simulink model "Task_No6_Thermal"  (R2023b)
settings: Solver=ode5  StartTime=0.0  StopTime=3600*24*7  FixedStep=1  RelTol=1e-3
InitFcn:
  | PARAMETERS;
StartFcn:
  | PARAMETERS;
values from neighbouring files (symbols this model uses):
  Conv_C_to_K = 273.15    [PARAMETERS.m]
  P_AC_AIR_FLOW = 1    [PARAMETERS.m]
  P_AREA_BATH = 2*4    (= 8)    [PARAMETERS.m]
  P_AREA_BDR1 = 3.87^2    (= 14.9769)    [PARAMETERS.m]
  P_AREA_BDR2 = 3.87*4.5    (= 17.415)    [PARAMETERS.m]
  P_AREA_EAST_WALL_BATH = 2*P_RM_HEIGHT - P_AREA_WIN_BATH    (= 3.7)    [PARAMETERS.m]
  P_AREA_EAST_WALL_BDR2 = 3.87*P_RM_HEIGHT - P_AREA_WIN_BDRS    (= 7.075)    [PARAMETERS.m]
  P_AREA_EAST_WALL_KIT = 4.13*P_RM_HEIGHT    (= 10.325)    [PARAMETERS.m]
  P_AREA_HALL = 2*6    (= 12)    [PARAMETERS.m]
  P_AREA_KIT = 4.13*4    (= 16.52)    [PARAMETERS.m]
  P_AREA_LVR = 4.13*6    (= 24.78)    [PARAMETERS.m]
  P_AREA_NORTH_WALL_BATH = 1.63*P_RM_HEIGHT    (= 4.075)    [PARAMETERS.m]
  P_AREA_NORTH_WALL_BDR1 = 3.87*P_RM_HEIGHT - P_AREA_WIN_BDRS    (= 7.075)    [PARAMETERS.m]
  P_AREA_NORTH_WALL_BDR2 = 4.5*P_RM_HEIGHT - P_AREA_WIN_BDRS    (= 8.65)    [PARAMETERS.m]
  P_AREA_OUTER_WALL_BATH = (1.63+2)*P_RM_HEIGHT - P_AREA_WIN_BATH    (= 7.775)    [PARAMETERS.m]
  P_AREA_OUTER_WALL_BDR1 = 3.87*2*P_RM_HEIGHT - P_AREA_WIN_BDRS    (= 16.75)    [PARAMETERS.m]
  P_AREA_OUTER_WALL_BDR2 = (4.5+3.87)*P_RM_HEIGHT - P_AREA_WIN_BDRS*2    (= 15.725)    [PARAMETERS.m]
  P_AREA_OUTER_WALL_HALL = 2*P_RM_HEIGHT - P_AREA_SING_DOOR    (= 2.9)    [PARAMETERS.m]
  P_AREA_OUTER_WALL_KIT = (4+4.13)*P_RM_HEIGHT - P_AREA_WIN_KIT    (= 13.725)    [PARAMETERS.m]
  P_AREA_OUTER_WALL_LVR = (4.13+6)*P_RM_HEIGHT - P_AREA_WIN_LVR    (= 14.325)    [PARAMETERS.m]
  P_AREA_SOUTH_WALL_KIT = 4*P_RM_HEIGHT - P_AREA_WIN_KIT    (= 3.4)    [PARAMETERS.m]
  P_AREA_SOUTH_WALL_LVR = 6*P_RM_HEIGHT - P_AREA_WIN_LVR    (= 4)    [PARAMETERS.m]
  P_AREA_WALL_BATH_KIT = 4*P_RM_HEIGHT    (= 10)    [PARAMETERS.m]
  P_AREA_WALL_BDR1_BDR2 = 3.87*P_RM_HEIGHT    (= 9.675)    [PARAMETERS.m]
  P_AREA_WALL_BDR1_HALL = 3.87*P_RM_HEIGHT - P_AREA_SING_DOOR    (= 7.575)    [PARAMETERS.m]
  P_AREA_WALL_BDR2_BATH = 2.37*P_RM_HEIGHT    (= 5.925)    [PARAMETERS.m]
  P_AREA_WALL_BDR2_HALL = 2.13*P_RM_HEIGHT - P_AREA_SING_DOOR    (= 3.225)    [PARAMETERS.m]
  P_AREA_WALL_HALL_BATH = 2*P_RM_HEIGHT - P_AREA_SING_DOOR    (= 2.9)    [PARAMETERS.m]
  P_AREA_WALL_HALL_LVR = 6*P_RM_HEIGHT - P_AREA_DBL_DOOR    (= 10.8)    [PARAMETERS.m]
  P_AREA_WALL_LVR_KIT = 4.13*P_RM_HEIGHT - P_AREA_DBL_DOOR    (= 6.125)    [PARAMETERS.m]
  P_AREA_WIN_BATH = P_H_WIN_NORM*P_W_WIN_BATH    (= 1.3)    [PARAMETERS.m]
  P_AREA_WIN_BDRS = P_H_WIN_NORM*P_W_WIN_BDRS    (= 2.6)    [PARAMETERS.m]
  P_AREA_WIN_KIT = P_H_WIN_DOOR*P_W_WIN_KIT    (= 6.6)    [PARAMETERS.m]
  P_AREA_WIN_LVR = P_H_WIN_DOOR*P_W_WIN_LVR    (= 11)    [PARAMETERS.m]
  P_CP_AIR = 1012    [PARAMETERS.m]
  P_DENSITY_BRICK = 2/(10^-3)    (= 2000)    [PARAMETERS.m]
  P_DENSITY_PUR = 150    [PARAMETERS.m]
  P_EM_GLASS = 0.94    [PARAMETERS.m]
  P_EM_WALL = 0.94    [PARAMETERS.m]
  P_HUMAN = 60    [PARAMETERS.m]
  P_M_WINDOW_SPEC = 20    [PARAMETERS.m]
  P_THICK_BRICK = 0.175    [PARAMETERS.m]
  P_THICK_PUR = P_THICK_WALL - P_THICK_BRICK    (= 0.125)    [PARAMETERS.m]
  T_COOLER = 12    [PARAMETERS.m]
  T_HEATER = 50    [PARAMETERS.m]
  T_INIT_BDR = 22    [PARAMETERS.m]
  T_INIT_OUT = 2.9    [PARAMETERS.m]
  U_CEIL = 1.1    [PARAMETERS.m]
  U_INNER_WALL_BR = 3    [PARAMETERS.m]
  U_INNER_WALL_PC = 0.6    [PARAMETERS.m]
  U_WALL = 0.32    [PARAMETERS.m]
  U_WINDOW = 3.0    (= 3)    [PARAMETERS.m]
undefined symbols (not defined in the file or in its folder): TBL_SOL_EAST_01, TBL_SOL_EAST_02, TBL_SOL_EAST_03, TBL_SOL_EAST_04, TBL_SOL_EAST_05, TBL_SOL_EAST_06, TBL_SOL_EAST_07, TBL_SOL_EAST_08, TBL_SOL_EAST_09, TBL_SOL_EAST_10, TBL_SOL_EAST_11, TBL_SOL_EAST_12, TBL_SOL_NORTH_01, TBL_SOL_NORTH_02, TBL_SOL_NORTH_03, TBL_SOL_NORTH_04, TBL_SOL_NORTH_05, TBL_SOL_NORTH_06, TBL_SOL_NORTH_07, TBL_SOL_NORTH_08, TBL_SOL_NORTH_09, TBL_SOL_NORTH_10, TBL_SOL_NORTH_11, TBL_SOL_NORTH_12, TBL_SOL_SOUTH_01, TBL_TEMP
libraries: fl_lib x135, nesl_utility x39, slpidlib x3
(part 1 of 3)
settings Model: Creator=Selim  LastModifiedBy=Selim

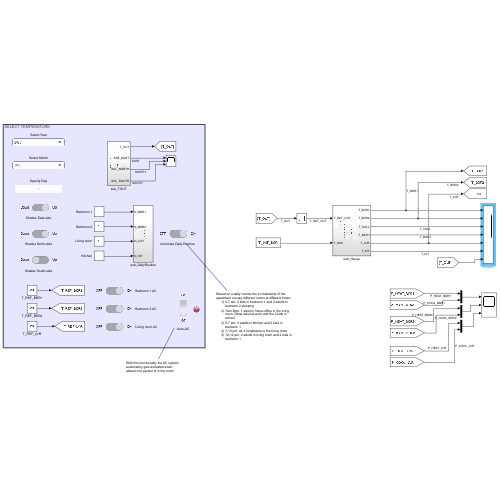
[thumbnail: Simulink's stored preview of the top-level diagram]
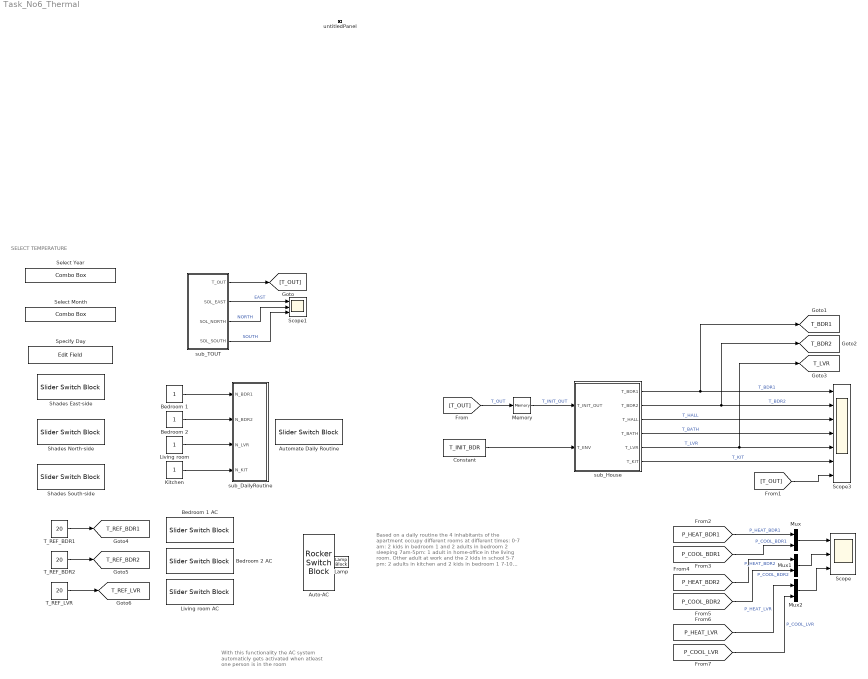
== system Task_No6_Thermal ==
  note: With this functionality the AC system automaticly gets activated when atleast one person is in the room
  note: SELECT TEMPERATURE
  note: Based on a daily routine the 4 inhabitants of the apartment occupy different rooms at different times:
      | 0-7 am: 2 kids in bedroom 1 and 2 adults in bedroom 2 sleeping
      | 7am-5pm: 1 adult in home-office in the living room. Other adult at work and the 2 kids in school
      | 5-7 pm: 2 adults in kitchen and 2 kids in bedroom 1
      | 7-10 pm: all 4 inhabitants in the living room
      | 10-12 pm: 2 adults in living room and 2 kids in bedroom 1
  Auto-AC : RockerSwitchBlock  LabelPosition=Hide
      settings: Values={{'Off', 'On'}, [0 1]}
  Automate Daily Routine : SliderSwitchBlock  LabelPosition=Hide
      settings: Values={{'OFF', 'ON'}, [0 1]}
  Bedroom 1 : Constant
  Bedroom 1 AC : SliderSwitchBlock  LabelPosition=Hide
      settings: Values={{'OFF', 'ON'}, [0 1]}
  Bedroom 2 : Constant
  Bedroom 2 AC : SliderSwitchBlock  LabelPosition=Hide
      settings: Values={{'OFF', 'ON'}, [0 1]}
  Constant : Constant  Value=T_INIT_BDR
  Kitchen : Constant
  Lamp : LampBlock  LabelPosition=Hide
  Living room : Constant
  Living room AC : SliderSwitchBlock  LabelPosition=Hide
      settings: Values={{'OFF', 'ON'}, [0 1]}
  Memory : Memory  InitialCondition=T_INIT_OUT
  Mux : Mux  Inputs=2
  Mux1 : Mux  Inputs=2
  Mux2 : Mux  Inputs=2
  Scope : Scope  NumInputPorts=3
  Scope1 : Scope  NumInputPorts=3
  Scope3 : Scope  NumInputPorts=7
  Select Month : ComboBox  LabelPosition=Hide  SelectedLabel=July
      settings: Values={{'January', 'February', 'March', 'April', 'May', 'June', 'July', 'August', 'September', 'Oktober', 'November', 'December'}, [1 2 3 4 5 6 7 8 9 10 11 12]}
  Select Year : ComboBox  LabelPosition=Hide  SelectedLabel=2023
      settings: Values={{'2022', '2023'}, [2022 2023]}
  Shades East-side : SliderSwitchBlock  LabelPosition=Hide
      settings: Values={{'Down', 'Up'}, [0 1]}
  Shades North-side : SliderSwitchBlock  LabelPosition=Hide
      settings: Values={{'Down', 'Up'}, [0 1]}
  Shades South-side : SliderSwitchBlock  LabelPosition=Hide
      settings: Values={{'Down', 'Up'}, [0 1]}
  Specify Day : EditField  LabelPosition=Hide  ShowInitialText=on  Alignment=Center
  T_REF_BDR1 : Constant  Value=20
  T_REF_BDR2 : Constant  Value=20
  T_REF_LVR : Constant  Value=20
  sub_DailyRoutine : Subsystem
  sub_House : Subsystem
  sub_TOUT : Subsystem
  untitledPanel : Subsystem  Tag=HiddenForWebPanel  IsWebBlockPanel=on
  tag scope: T_BDR1=global, T_BDR2=global, T_LVR=global, T_REF_BDR1=global, T_REF_BDR2=global, T_REF_LVR=global
  wires:
  Memory/1 -> sub_House/1(T_INIT_OUT)  "T_INIT_OUT"
  sub_House/1(T_BDR1) -> [T_BDR1], Scope3/1  "T_BDR1"
  [T_OUT] -> Memory/1  "T_OUT"
  [T_OUT] -> Scope3/7
  Constant/1 -> sub_House/2(T_ENV)
  sub_TOUT/1(T_OUT) -> [T_OUT]
  sub_House/2(T_BDR2) -> [T_BDR2], Scope3/2  "T_BDR2"
  sub_House/3(T_HALL) -> Scope3/3  "T_HALL"
  sub_House/4(T_BATH) -> Scope3/4  "T_BATH"
  sub_House/5(T_LVR) -> [T_LVR], Scope3/5  "T_LVR"
  sub_House/6(T_KIT) -> Scope3/6  "T_KIT"
  sub_TOUT/2(SOL_EAST) -> Scope1/1  "EAST"
  sub_TOUT/3(SOL_NORTH) -> Scope1/2  "NORTH"
  sub_TOUT/4(SOL_SOUTH) -> Scope1/3  "SOUTH"
  Bedroom 1/1 -> sub_DailyRoutine/1(N_BDR1)
  Bedroom 2/1 -> sub_DailyRoutine/2(N_BDR2)
  Living room/1 -> sub_DailyRoutine/3(N_LVR)
  Kitchen/1 -> sub_DailyRoutine/4(N_KIT)
  T_REF_BDR1/1 -> [T_REF_BDR1]
  T_REF_BDR2/1 -> [T_REF_BDR2]
  T_REF_LVR/1 -> [T_REF_LVR]
  Mux/1 -> Scope/1
  Mux1/1 -> Scope/2
  Mux2/1 -> Scope/3
  [P_HEAT_BDR1] -> Mux/1  "P_HEAT_BDR1"
  [P_COOL_BDR1] -> Mux/2  "P_COOL_BDR1"
  [P_HEAT_BDR2] -> Mux1/1  "P_HEAT_BDR2"
  [P_COOL_BDR2] -> Mux1/2  "P_COOL_BDR2"
  [P_HEAT_LVR] -> Mux2/1  "P_HEAT_LVR"
  [P_COOL_LVR] -> Mux2/2  "P_COOL_LVR"

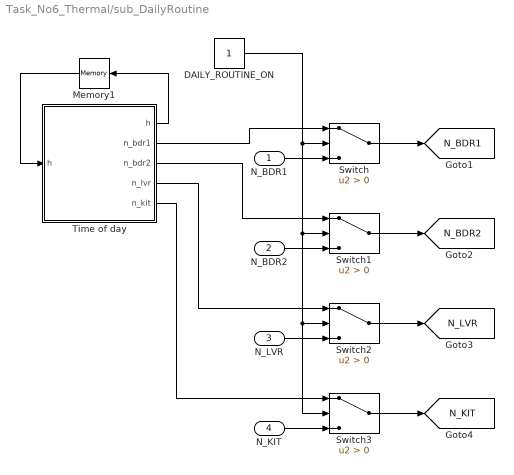
== system Task_No6_Thermal/sub_DailyRoutine ==
  N_BDR1 : Inport
  N_BDR2 : Inport  Port=2
  N_LVR : Inport  Port=3
  N_KIT : Inport  Port=4
  DAILY_ROUTINE_ON : Constant
  Memory1 : Memory
  Switch{,1..3} (4 alike) : Switch  Criteria=u2 > Threshold  SaturateOnIntegerOverflow=off  InputSameDT=off
  Time of day : MATLAB Function  TreatAsAtomicUnit=on
  tag scope: N_BDR1=global, N_BDR2=global, N_KIT=global, N_LVR=global
  wires:
  Switch1/1 -> [N_BDR2]
  Switch2/1 -> [N_LVR]
  Time of day/1(h) -> Memory1/1
  Memory1/1 -> Time of day/1("h ")
  Switch/1 -> [N_BDR1]
  Switch3/1 -> [N_KIT]
  Time of day/2(n_bdr1) -> Switch/1
  Time of day/3(n_bdr2) -> Switch1/1
  Time of day/4(n_lvr) -> Switch2/1
  Time of day/5(n_kit) -> Switch3/1
  DAILY_ROUTINE_ON/1 -> Switch3/2, Switch2/2, Switch1/2, Switch/2
  N_BDR1/1 -> Switch/3
  N_BDR2/1 -> Switch1/3
  N_LVR/1 -> Switch2/3
  N_KIT/1 -> Switch3/3

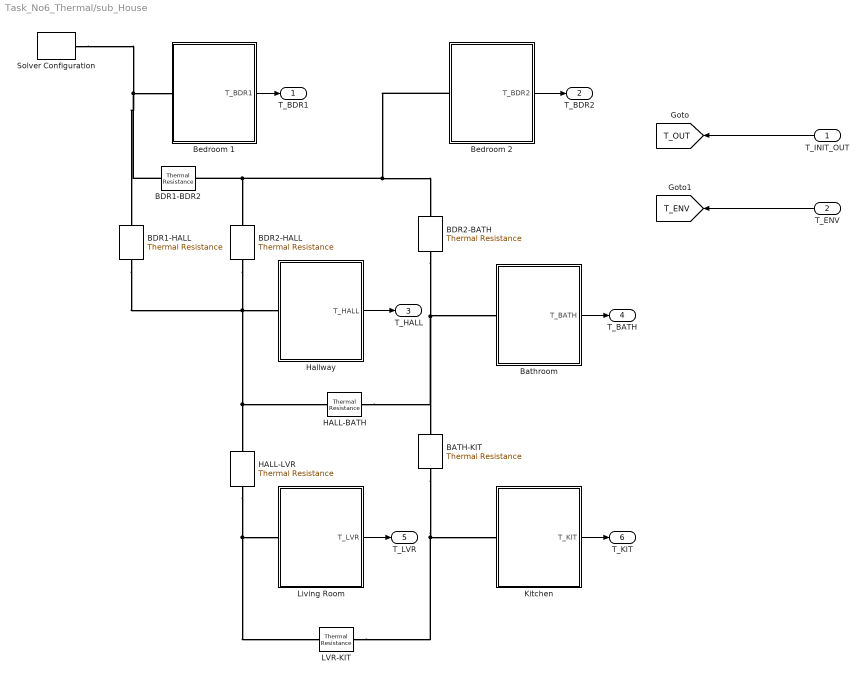
== system Task_No6_Thermal/sub_House ==
  T_INIT_OUT : Inport
  T_ENV : Inport  Port=2
  BATH-KIT : fl_lib/Thermal/Thermal Elements/Thermal Resistance  resistance=1/(U_INNER_WALL_PC*P_AREA_WALL_BATH_KIT) K/W  T_specify=off  T_priority=None  T=0 K  T_nominal_specify=off  T_nominal_unit=K  T_nominal_value=1  Q_specify=off  Q_priority=None  Q=0 W  Q_nominal_specify=off  Q_nominal_unit=W  Q_nominal_value=1
  BDR1-BDR2 : fl_lib/Thermal/Thermal Elements/Thermal Resistance  resistance=1/(U_INNER_WALL_BR*P_AREA_WALL_BDR1_BDR2) K/W  T_specify=off  T_priority=None  T=0 K  T_nominal_specify=off  T_nominal_unit=K  T_nominal_value=1  Q_specify=off  Q_priority=None  Q=0 W  Q_nominal_specify=off  Q_nominal_unit=W  Q_nominal_value=1
  BDR1-HALL : fl_lib/Thermal/Thermal Elements/Thermal Resistance  resistance=1/(U_INNER_WALL_PC*P_AREA_WALL_BDR1_HALL) K/W  T_specify=off  T_priority=None  T=0 K  T_nominal_specify=off  T_nominal_unit=K  T_nominal_value=1  Q_specify=off  Q_priority=None  Q=0 W  Q_nominal_specify=off  Q_nominal_unit=W  Q_nominal_value=1
  BDR2-BATH : fl_lib/Thermal/Thermal Elements/Thermal Resistance  resistance=1/(U_INNER_WALL_PC*P_AREA_WALL_BDR2_BATH) K/W  T_specify=off  T_priority=None  T=0 K  T_nominal_specify=off  T_nominal_unit=K  T_nominal_value=1  Q_specify=off  Q_priority=None  Q=0 W  Q_nominal_specify=off  Q_nominal_unit=W  Q_nominal_value=1
  BDR2-HALL : fl_lib/Thermal/Thermal Elements/Thermal Resistance  resistance=1/(U_INNER_WALL_PC*P_AREA_WALL_BDR2_HALL) K/W  T_specify=off  T_priority=None  T=0 K  T_nominal_specify=off  T_nominal_unit=K  T_nominal_value=1  Q_specify=off  Q_priority=None  Q=0 W  Q_nominal_specify=off  Q_nominal_unit=W  Q_nominal_value=1
  Bathroom : Subsystem
  Bedroom 1 : Subsystem
  Bedroom 2 : Subsystem
  HALL-BATH : fl_lib/Thermal/Thermal Elements/Thermal Resistance  resistance=1/(U_INNER_WALL_BR*P_AREA_WALL_HALL_BATH) K/W  T_specify=off  T_priority=None  T=0 K  T_nominal_specify=off  T_nominal_unit=K  T_nominal_value=1  Q_specify=off  Q_priority=None  Q=0 W  Q_nominal_specify=off  Q_nominal_unit=W  Q_nominal_value=1
  HALL-LVR : fl_lib/Thermal/Thermal Elements/Thermal Resistance  resistance=1/(U_INNER_WALL_PC*P_AREA_WALL_HALL_LVR) K/W  T_specify=off  T_priority=None  T=0 K  T_nominal_specify=off  T_nominal_unit=K  T_nominal_value=1  Q_specify=off  Q_priority=None  Q=0 W  Q_nominal_specify=off  Q_nominal_unit=W  Q_nominal_value=1
  Hallway : Subsystem
  Kitchen : Subsystem
  LVR-KIT : fl_lib/Thermal/Thermal Elements/Thermal Resistance  resistance=1/(U_INNER_WALL_BR*P_AREA_WALL_LVR_KIT) K/W  T_specify=off  T_priority=None  T=0 K  T_nominal_specify=off  T_nominal_unit=K  T_nominal_value=1  Q_specify=off  Q_priority=None  Q=0 W  Q_nominal_specify=off  Q_nominal_unit=W  Q_nominal_value=1
  Living Room : Subsystem
  Solver Configuration : nesl_utility/Solver Configuration  PhysicalDomain=network_engine_domain  SubClassName=solver  LeftPortType=input  RightPortType=generic  Tones=[]  Harmonics=[]  SimulateNoise=off  Profile=off  UseLocalSampling=off  EnableSwitchedLinearOptims=on  FrequencyDomain=off  UseCCode=off  RelTol=0.001  AbsTol=0.001  MinStep=1e-09  ToWorkspace=off  RevertToSquareIcSolve=off  NumHomotopyIterations=100  PhasorMode=off  PhasorModeNumHarmonics=1  ConsistencySolver=NEWTON_XTOL_AFTER_FTOL  IndexReductionMethod=DerivativeReplacement  DoDC=off  ResidualTolerance=1e-09  ConsistencyTolSource=GLOBAL  ConsistencyAbsTol=0.001  ConsistencyRelTol=0.001  ConsistencyTolFactor=0.001  UseLocalSolver=off  LocalSolverChoice=NE_BACKWARD_EULER_ADVANCER  ResolveIndetEquations=on  FunctionEvalNumThread=1  LocalSolverSampleTime=0.001  DoFixedCost=off  MaxNonlinIter=3  MaxModeIter=2  ComputeImpulses=off  ImpulseIterations=2  LinearAlgebra=auto  LinearAlgebraNumThread=0  EquationFormulation=NE_TIME_EF  DelaysMemoryBudget=1024  AutomaticFiltering=on  FilteringTimeConstant=0.001  PartitionStorageMethod=AS_NEEDED  PartitionMemoryBudget=1024  PartitionMethod=ROBUST  MultibodyUseLocalSolver=off  MultibodyLocalSolverChoice=ODE1  MultibodyLocalSolverSampleTime=0.001
  T_BDR1 : Outport
  T_BDR2 : Outport  Port=2
  T_HALL : Outport  Port=3
  T_BATH : Outport  Port=4
  T_LVR : Outport  Port=5
  T_KIT : Outport  Port=6
  tag scope: T_ENV=global, T_OUT=global
  wires:
  Bedroom 1/1(T_BDR1) -> T_BDR1/1
  T_INIT_OUT/1 -> [T_OUT]
  T_ENV/1 -> [T_ENV]
  Bedroom 2/1(T_BDR2) -> T_BDR2/1
  Hallway/1(T_HALL) -> T_HALL/1
  Bathroom/1(T_BATH) -> T_BATH/1
  Living Room/1(T_LVR) -> T_LVR/1
  Kitchen/1(T_KIT) -> T_KIT/1
  connections:
  Solver Configuration/RConn1 -- BDR1-HALL/LConn1 -- BDR1-BDR2/RConn1 -- Bedroom 1/LConn1
  Bedroom 2/LConn1 -- BDR2-BATH/LConn1 -- BDR2-HALL/LConn1 -- BDR1-BDR2/LConn1
  BDR2-BATH/RConn1 -- HALL-BATH/LConn1 -- BATH-KIT/LConn1 -- Bathroom/LConn1
  BATH-KIT/RConn1 -- LVR-KIT/LConn1 -- Kitchen/LConn1
  HALL-LVR/RConn1 -- Living Room/LConn1 -- LVR-KIT/RConn1
  BDR1-HALL/RConn1 -- HALL-LVR/LConn1 -- HALL-BATH/RConn1 -- Hallway/LConn1 -- BDR2-HALL/RConn1

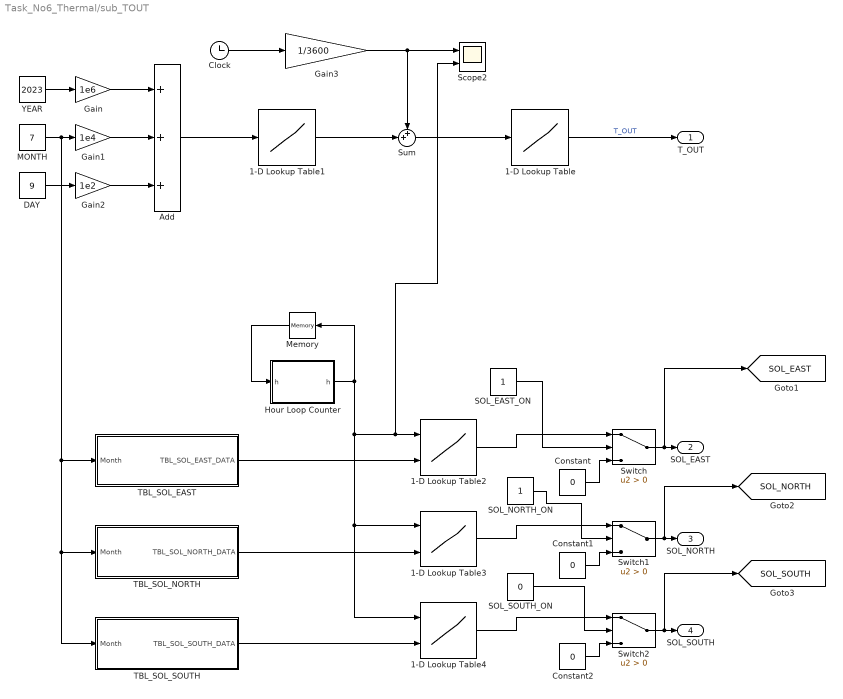
== system Task_No6_Thermal/sub_TOUT ==
  1-D Lookup Table : Lookup_n-D  NumberOfTableDimensions=1  BreakpointsForDimension1=TBL_TEMP.DATE_sec  Table=TBL_TEMP.T_C  InternalRulePriority=Speed  RndMeth=Simplest
  1-D Lookup Table1 : Lookup_n-D  NumberOfTableDimensions=1  BreakpointsForDimension1=TBL_TEMP.DATE_yyyymmddhh  Table=TBL_TEMP.DATE_sec  InternalRulePriority=Speed  RndMeth=Simplest
  1-D Lookup Table2 : Lookup_n-D  NumberOfTableDimensions=1  BreakpointsForDimension1=0:1:23  TableSource=Input port  Table=tanh([-5:5])  InternalRulePriority=Speed  RndMeth=Simplest
      settings: InputPortMap=u0,p221
  1-D Lookup Table3 : Lookup_n-D  NumberOfTableDimensions=1  BreakpointsForDimension1=0:1:23  TableSource=Input port  Table=tanh([-5:5])  InternalRulePriority=Speed  RndMeth=Simplest
      settings: InputPortMap=u0,p221
  1-D Lookup Table4 : Lookup_n-D  NumberOfTableDimensions=1  BreakpointsForDimension1=0:1:23  TableSource=Input port  Table=tanh([-5:5])  InternalRulePriority=Speed  RndMeth=Simplest
      settings: InputPortMap=u0,p221
  Add : Sum  Inputs=+++
  Clock : Clock
  Constant : Constant  Value=0
  Constant1 : Constant  Value=0
  Constant2 : Constant  Value=0
  DAY : Constant  Value=9
  Gain : Gain  Gain=1e6
  Gain1 : Gain  Gain=1e4
  Gain2 : Gain  Gain=1e2
  Gain3 : Gain  Gain=1/3600
  Hour Loop Counter : MATLAB Function  TreatAsAtomicUnit=on
  MONTH : Constant  Value=7
  Memory : Memory
  SOL_EAST_ON : Constant
  SOL_NORTH_ON : Constant
  SOL_SOUTH_ON : Constant  Value=0
  Scope2 : Scope  NumInputPorts=2
  Sum : Sum  Inputs=++|
  Switch : Switch  Criteria=u2 > Threshold  SaturateOnIntegerOverflow=off  InputSameDT=off
  Switch1 : Switch  Criteria=u2 > Threshold  SaturateOnIntegerOverflow=off  InputSameDT=off
  Switch2 : Switch  Criteria=u2 > Threshold  SaturateOnIntegerOverflow=off  InputSameDT=off
  TBL_SOL_EAST : Subsystem
  TBL_SOL_NORTH : Subsystem
  TBL_SOL_SOUTH : Subsystem
  YEAR : Constant  Value=2023
  T_OUT : Outport
  SOL_EAST : Outport  Port=2
  SOL_NORTH : Outport  Port=3
  SOL_SOUTH : Outport  Port=4
  tag scope: SOL_EAST=global, SOL_NORTH=global, SOL_SOUTH=global
  wires:
  Gain1/1 -> Add/2
  MONTH/1 -> TBL_SOL_SOUTH/1(Month), TBL_SOL_NORTH/1(Month), TBL_SOL_EAST/1(Month), Gain1/1
  Clock/1 -> Gain3/1
  1-D Lookup Table1/1 -> Sum/2
  Add/1 -> 1-D Lookup Table1/1
  YEAR/1 -> Gain/1
  Gain/1 -> Add/1
  Gain3/1 -> Scope2/1, Sum/1
  Sum/1 -> 1-D Lookup Table/1
  Gain2/1 -> Add/3
  DAY/1 -> Gain2/1
  1-D Lookup Table/1 -> T_OUT/1  "T_OUT"
  Hour Loop Counter/1(h) -> 1-D Lookup Table4/1, 1-D Lookup Table3/1, Scope2/2, 1-D Lookup Table2/1, Memory/1
  Memory/1 -> Hour Loop Counter/1("h ")
  Switch/1 -> [SOL_EAST], SOL_EAST/1
  TBL_SOL_EAST/1(TBL_SOL_EAST_DATA) -> 1-D Lookup Table2/2
  TBL_SOL_NORTH/1(TBL_SOL_NORTH_DATA) -> 1-D Lookup Table3/2
  TBL_SOL_SOUTH/1(TBL_SOL_SOUTH_DATA) -> 1-D Lookup Table4/2
  Switch1/1 -> [SOL_NORTH], SOL_NORTH/1
  Switch2/1 -> [SOL_SOUTH], SOL_SOUTH/1
  1-D Lookup Table2/1 -> Switch/1
  1-D Lookup Table3/1 -> Switch1/1
  1-D Lookup Table4/1 -> Switch2/1
  SOL_EAST_ON/1 -> Switch/2
  Constant/1 -> Switch/3
  Constant1/1 -> Switch1/3
  Constant2/1 -> Switch2/3
  SOL_NORTH_ON/1 -> Switch1/2
  SOL_SOUTH_ON/1 -> Switch2/2

== system Task_No6_Thermal/untitledPanel ==
  Radio Button : RadioButtonGroup  Tag=HiddenForWebPanel  PanelInfo="{\"addnFilesFolder\":\"\",\"height\":230,\"includeDebugPackages\":false,\"left\":18,\"outputFolder\":\"\",\"panelId\":\"panelId-a10107d6-1e7d-451d-956e-0df6eada92c1\",\"popoutMode\":\"\",\"standaloneTitle\":\"\",\"top\":18,\"type\":\"panelChild\",\"version\":\"2019b\",\"width\":270,\"zIndex\":1500002}"  SelectedLabel=Label3  ButtonGroupName=Group
      settings: Values={{'Label1', 'Label2', 'Label3'}, [0 1 2]}
  panelInfo : PanelWebBlock  Tag=HiddenForWebPanel  PanelInfo="{\"addnFilesFolder\":\"\",\"compacted\":false,\"height\":270,\"includeDebugPackages\":false,\"isActiveTab\":true,\"left\":296,\"name\":\"Panel\",\"outputFolder\":\"\",\"panelId\":\"panelId-a10107d6-1e7d-451d-956e-0df6eada92c1\",\"popoutData\":{\"height\":334,\"left\":361,\"maximized\":false,\"top\":306,\"width\":324},\"popoutMode\":\"windowHidden\",\"standaloneTitle\":\"\",\"tabIndex\":0,\"tabbedSetId\":\"tabbedSet8433950298\",\"top\":135,\"type\":\"panel\",\"version\":\"2019b\",\"visible\":true,\"width\":310,\"zIndex\":1500002}"

== system Task_No6_Thermal/sub_House/Bathroom ==
  Ceiling & Floor (Bath<->Above & Below) : Subsystem
  Inside Enivornment Temperature : Subsystem
      settings: PortSchema="{\"entries\":[{\"content\":{\"sides\":[{\"content\":{\"connectorIds\":[\"LConn1\"]},\"type\":\"ConnectorPlacement.EquallySpacedRectSide\",\"uuid\":\"d7207a88-d4d1-4eb1-8525-bfbf38cfed80\"},{\"content\":{\"connectorIds\":[\"In1\"],\"side\":\"RIGHT\"},\"type\":\"ConnectorPlacement.EquallySpacedRectSide\",\"uuid\":\"a5beddf3-616c-4e89-970e-855bf6dc3854\"},{\"content\":{\"side\":\"TOP\"},\"type\":\"ConnectorPlacement.EquallySpacedRectSide\",\"uuid\":\"3f9b2b25-be8a-4286-a049-e39ed58f5b46\"}]},\"type\":\"ConnectorPlacement.EquallySpacedConnector\",\"uuid\":\"525311df-b3f4-411a-b576-8112a1b0b63b\"}],\"packageUris\":[\"http://schema.mathworks.com/mf0/Connector/R2020b\"],\"version\":\"1.0\"}"
  Outside Temperature : Subsystem
      settings: PortSchema="{\"entries\":[{\"content\":{\"sides\":[{\"content\":{\"connectorIds\":[\"LConn1\"]},\"type\":\"ConnectorPlacement.EquallySpacedRectSide\",\"uuid\":\"d7207a88-d4d1-4eb1-8525-bfbf38cfed80\"},{\"content\":{\"connectorIds\":[\"In1\"],\"side\":\"RIGHT\"},\"type\":\"ConnectorPlacement.EquallySpacedRectSide\",\"uuid\":\"a5beddf3-616c-4e89-970e-855bf6dc3854\"},{\"content\":{\"side\":\"TOP\"},\"type\":\"ConnectorPlacement.EquallySpacedRectSide\",\"uuid\":\"3f9b2b25-be8a-4286-a049-e39ed58f5b46\"}]},\"type\":\"ConnectorPlacement.EquallySpacedConnector\",\"uuid\":\"525311df-b3f4-411a-b576-8112a1b0b63b\"}],\"packageUris\":[\"http://schema.mathworks.com/mf0/Connector/R2020b\"],\"version\":\"1.0\"}"
  SOLAR__WALL : Subsystem
  SOLAR__WINDOW : Subsystem
  TEMP_01 : Subsystem
  Thermal Mass of inside air : fl_lib/Thermal/Thermal Elements/Thermal Mass  mass_type=foundation.enum.constant_variable.constant  mass=P_M_AIR_BATH kg  sp_heat=P_CP_AIR J/(K*kg)  mass_min=1e-6 kg  num_ports=foundation.enum.numPorts2.one  m_specify=off  m_priority=High  m=1 kg  m_nominal_specify=off  m_nominal_unit=kg  m_nominal_value=1  T_specify=on  T_priority=High  T=T_INIT_BDR degC  T_nominal_specify=off  T_nominal_unit=K  T_nominal_value=1  Q_specify=off  Q_priority=None  Q=0 W  Q_nominal_specify=off  Q_nominal_unit=W  Q_nominal_value=1
  Wall (Bath<->Outside) : Subsystem
  Window (Bath<->Outside) : Subsystem
  Conn1 : PMIOPort  Side=Left
  T_BATH : Outport
  wires:
  TEMP_01/1(Sim) -> T_BATH/1
  [T_OUT] -> Outside Temperature/1(T_OUT)
  [T_ENV] -> Inside Enivornment Temperature/1(T_ENV)
  connections:
  Window (Bath<->Outside)/RConn1 -- Outside Temperature/LConn1 -- Wall (Bath<->Outside)/RConn2
  TEMP_01/LConn1 -- Conn1/RConn1 -- Wall (Bath<->Outside)/LConn1 -- Thermal Mass of inside air/LConn1 -- Window (Bath<->Outside)/LConn1 -- Ceiling & Floor (Bath<->Above & Below)/RConn1
  Inside Enivornment Temperature/LConn1 -- Ceiling & Floor (Bath<->Above & Below)/LConn1
  SOLAR__WALL/LConn1 -- Wall (Bath<->Outside)/RConn1
  SOLAR__WINDOW/LConn1 -- Window (Bath<->Outside)/RConn2

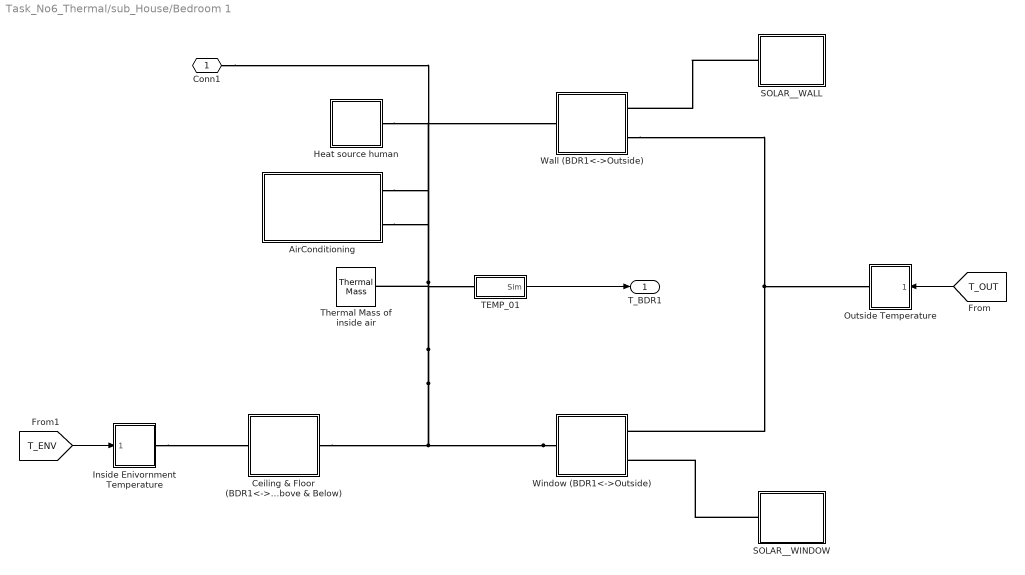
== system Task_No6_Thermal/sub_House/Bedroom 1 ==
  AirConditioning : Subsystem
  Ceiling & Floor (BDR1<->Above & Below) : Subsystem
  Heat source human : Subsystem
  Inside Enivornment Temperature : Subsystem
      settings: PortSchema="{\"entries\":[{\"content\":{\"sides\":[{\"content\":{\"connectorIds\":[\"LConn1\"]},\"type\":\"ConnectorPlacement.EquallySpacedRectSide\",\"uuid\":\"d7207a88-d4d1-4eb1-8525-bfbf38cfed80\"},{\"content\":{\"connectorIds\":[\"In1\"],\"side\":\"RIGHT\"},\"type\":\"ConnectorPlacement.EquallySpacedRectSide\",\"uuid\":\"a5beddf3-616c-4e89-970e-855bf6dc3854\"},{\"content\":{\"side\":\"TOP\"},\"type\":\"ConnectorPlacement.EquallySpacedRectSide\",\"uuid\":\"3f9b2b25-be8a-4286-a049-e39ed58f5b46\"}]},\"type\":\"ConnectorPlacement.EquallySpacedConnector\",\"uuid\":\"525311df-b3f4-411a-b576-8112a1b0b63b\"}],\"packageUris\":[\"http://schema.mathworks.com/mf0/Connector/R2020b\"],\"version\":\"1.0\"}"
  Outside Temperature : Subsystem
      settings: PortSchema="{\"entries\":[{\"content\":{\"sides\":[{\"content\":{\"connectorIds\":[\"LConn1\"]},\"type\":\"ConnectorPlacement.EquallySpacedRectSide\",\"uuid\":\"d7207a88-d4d1-4eb1-8525-bfbf38cfed80\"},{\"content\":{\"connectorIds\":[\"In1\"],\"side\":\"RIGHT\"},\"type\":\"ConnectorPlacement.EquallySpacedRectSide\",\"uuid\":\"a5beddf3-616c-4e89-970e-855bf6dc3854\"},{\"content\":{\"side\":\"TOP\"},\"type\":\"ConnectorPlacement.EquallySpacedRectSide\",\"uuid\":\"3f9b2b25-be8a-4286-a049-e39ed58f5b46\"}]},\"type\":\"ConnectorPlacement.EquallySpacedConnector\",\"uuid\":\"525311df-b3f4-411a-b576-8112a1b0b63b\"}],\"packageUris\":[\"http://schema.mathworks.com/mf0/Connector/R2020b\"],\"version\":\"1.0\"}"
  SOLAR__WALL : Subsystem
  SOLAR__WINDOW : Subsystem
  TEMP_01 : Subsystem
  Thermal Mass of inside air : fl_lib/Thermal/Thermal Elements/Thermal Mass  mass_type=foundation.enum.constant_variable.constant  mass=P_M_AIR_BDR1 kg  sp_heat=P_CP_AIR J/(K*kg)  mass_min=1e-6 kg  num_ports=foundation.enum.numPorts2.one  m_specify=off  m_priority=High  m=1 kg  m_nominal_specify=off  m_nominal_unit=kg  m_nominal_value=1  T_specify=on  T_priority=High  T=T_INIT_BDR degC  T_nominal_specify=off  T_nominal_unit=K  T_nominal_value=1  Q_specify=off  Q_priority=None  Q=0 W  Q_nominal_specify=off  Q_nominal_unit=W  Q_nominal_value=1
  Wall (BDR1<->Outside) : Subsystem
  Window (BDR1<->Outside) : Subsystem
  Conn1 : PMIOPort  Side=Left
  T_BDR1 : Outport
  wires:
  TEMP_01/1(Sim) -> T_BDR1/1
  [T_OUT] -> Outside Temperature/1(T_OUT)
  [T_ENV] -> Inside Enivornment Temperature/1(T_ENV)
  connections:
  Wall (BDR1<->Outside)/RConn2 -- Outside Temperature/LConn1 -- Window (BDR1<->Outside)/RConn1
  Window (BDR1<->Outside)/LConn1 -- TEMP_01/LConn1 -- AirConditioning/RConn2 -- AirConditioning/RConn1 -- Heat source human/LConn1 -- Conn1/RConn1 -- Wall (BDR1<->Outside)/LConn1 -- Thermal Mass of inside air/LConn1 -- Ceiling & Floor (BDR1<->Above & Below)/RConn1
  Inside Enivornment Temperature/LConn1 -- Ceiling & Floor (BDR1<->Above & Below)/LConn1
  SOLAR__WALL/LConn1 -- Wall (BDR1<->Outside)/RConn1
  SOLAR__WINDOW/LConn1 -- Window (BDR1<->Outside)/RConn2

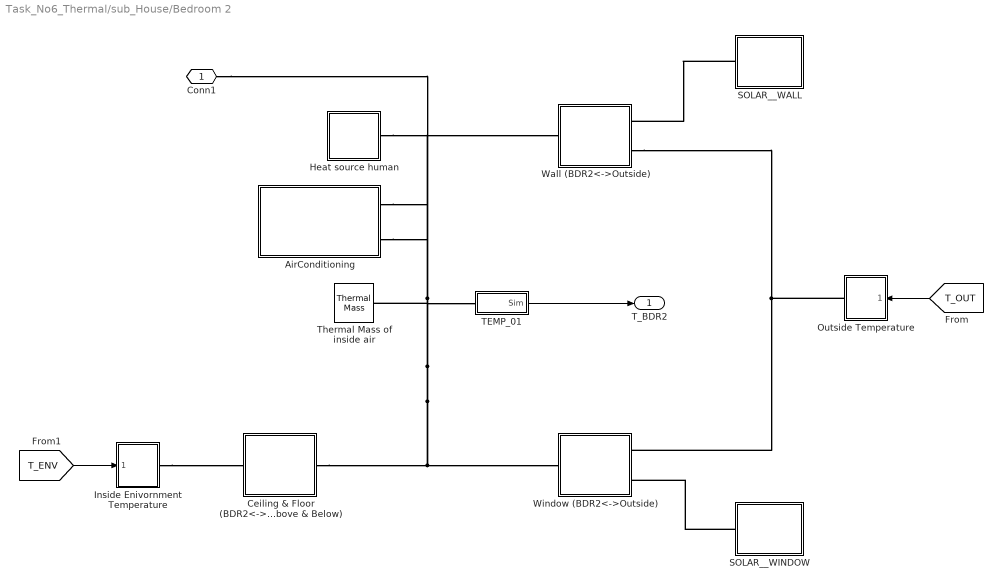
== system Task_No6_Thermal/sub_House/Bedroom 2 ==
  AirConditioning : Subsystem
  Ceiling & Floor (BDR2<->Above & Below) : Subsystem
  Heat source human : Subsystem
  Inside Enivornment Temperature : Subsystem
      settings: PortSchema="{\"entries\":[{\"content\":{\"sides\":[{\"content\":{\"connectorIds\":[\"LConn1\"]},\"type\":\"ConnectorPlacement.EquallySpacedRectSide\",\"uuid\":\"d7207a88-d4d1-4eb1-8525-bfbf38cfed80\"},{\"content\":{\"connectorIds\":[\"In1\"],\"side\":\"RIGHT\"},\"type\":\"ConnectorPlacement.EquallySpacedRectSide\",\"uuid\":\"a5beddf3-616c-4e89-970e-855bf6dc3854\"},{\"content\":{\"side\":\"TOP\"},\"type\":\"ConnectorPlacement.EquallySpacedRectSide\",\"uuid\":\"3f9b2b25-be8a-4286-a049-e39ed58f5b46\"}]},\"type\":\"ConnectorPlacement.EquallySpacedConnector\",\"uuid\":\"525311df-b3f4-411a-b576-8112a1b0b63b\"}],\"packageUris\":[\"http://schema.mathworks.com/mf0/Connector/R2020b\"],\"version\":\"1.0\"}"
  Outside Temperature : Subsystem
      settings: PortSchema="{\"entries\":[{\"content\":{\"sides\":[{\"content\":{\"connectorIds\":[\"LConn1\"]},\"type\":\"ConnectorPlacement.EquallySpacedRectSide\",\"uuid\":\"d7207a88-d4d1-4eb1-8525-bfbf38cfed80\"},{\"content\":{\"connectorIds\":[\"In1\"],\"side\":\"RIGHT\"},\"type\":\"ConnectorPlacement.EquallySpacedRectSide\",\"uuid\":\"a5beddf3-616c-4e89-970e-855bf6dc3854\"},{\"content\":{\"side\":\"TOP\"},\"type\":\"ConnectorPlacement.EquallySpacedRectSide\",\"uuid\":\"3f9b2b25-be8a-4286-a049-e39ed58f5b46\"}]},\"type\":\"ConnectorPlacement.EquallySpacedConnector\",\"uuid\":\"525311df-b3f4-411a-b576-8112a1b0b63b\"}],\"packageUris\":[\"http://schema.mathworks.com/mf0/Connector/R2020b\"],\"version\":\"1.0\"}"
  SOLAR__WALL : Subsystem
  SOLAR__WINDOW : Subsystem
  TEMP_01 : Subsystem
  Thermal Mass of inside air : fl_lib/Thermal/Thermal Elements/Thermal Mass  mass_type=foundation.enum.constant_variable.constant  mass=P_M_AIR_BDR2 kg  sp_heat=P_CP_AIR J/(K*kg)  mass_min=1e-6 kg  num_ports=foundation.enum.numPorts2.one  m_specify=off  m_priority=High  m=1 kg  m_nominal_specify=off  m_nominal_unit=kg  m_nominal_value=1  T_specify=on  T_priority=High  T=T_INIT_BDR degC  T_nominal_specify=off  T_nominal_unit=K  T_nominal_value=1  Q_specify=off  Q_priority=None  Q=0 W  Q_nominal_specify=off  Q_nominal_unit=W  Q_nominal_value=1
  Wall (BDR2<->Outside) : Subsystem
  Window (BDR2<->Outside) : Subsystem
  Conn1 : PMIOPort  Side=Left
  T_BDR2 : Outport
  wires:
  TEMP_01/1(Sim) -> T_BDR2/1
  [T_OUT] -> Outside Temperature/1(T_OUT)
  [T_ENV] -> Inside Enivornment Temperature/1(T_ENV)
  connections:
  Inside Enivornment Temperature/LConn1 -- Ceiling & Floor (BDR2<->Above & Below)/LConn1
  Ceiling & Floor (BDR2<->Above & Below)/RConn1 -- Window (BDR2<->Outside)/LConn1 -- Thermal Mass of inside air/LConn1 -- AirConditioning/RConn2 -- AirConditioning/RConn1 -- Heat source human/LConn1 -- Wall (BDR2<->Outside)/LConn1 -- Conn1/RConn1 -- TEMP_01/LConn1
  Wall (BDR2<->Outside)/RConn2 -- Outside Temperature/LConn1 -- Window (BDR2<->Outside)/RConn1
  SOLAR__WALL/LConn1 -- Wall (BDR2<->Outside)/RConn1
  SOLAR__WINDOW/LConn1 -- Window (BDR2<->Outside)/RConn2

== system Task_No6_Thermal/sub_House/Hallway ==
  Ceiling & Floor (Hall<->Above & Below) : Subsystem
  Inside Enivornment Temperature : Subsystem
      settings: PortSchema="{\"entries\":[{\"content\":{\"sides\":[{\"content\":{\"connectorIds\":[\"LConn1\"]},\"type\":\"ConnectorPlacement.EquallySpacedRectSide\",\"uuid\":\"d7207a88-d4d1-4eb1-8525-bfbf38cfed80\"},{\"content\":{\"connectorIds\":[\"In1\"],\"side\":\"RIGHT\"},\"type\":\"ConnectorPlacement.EquallySpacedRectSide\",\"uuid\":\"a5beddf3-616c-4e89-970e-855bf6dc3854\"},{\"content\":{\"side\":\"TOP\"},\"type\":\"ConnectorPlacement.EquallySpacedRectSide\",\"uuid\":\"3f9b2b25-be8a-4286-a049-e39ed58f5b46\"}]},\"type\":\"ConnectorPlacement.EquallySpacedConnector\",\"uuid\":\"525311df-b3f4-411a-b576-8112a1b0b63b\"}],\"packageUris\":[\"http://schema.mathworks.com/mf0/Connector/R2020b\"],\"version\":\"1.0\"}"
  Outside Temperature : Subsystem
      settings: PortSchema="{\"entries\":[{\"content\":{\"sides\":[{\"content\":{\"connectorIds\":[\"LConn1\"]},\"type\":\"ConnectorPlacement.EquallySpacedRectSide\",\"uuid\":\"d7207a88-d4d1-4eb1-8525-bfbf38cfed80\"},{\"content\":{\"connectorIds\":[\"In1\"],\"side\":\"RIGHT\"},\"type\":\"ConnectorPlacement.EquallySpacedRectSide\",\"uuid\":\"a5beddf3-616c-4e89-970e-855bf6dc3854\"},{\"content\":{\"side\":\"TOP\"},\"type\":\"ConnectorPlacement.EquallySpacedRectSide\",\"uuid\":\"3f9b2b25-be8a-4286-a049-e39ed58f5b46\"}]},\"type\":\"ConnectorPlacement.EquallySpacedConnector\",\"uuid\":\"525311df-b3f4-411a-b576-8112a1b0b63b\"}],\"packageUris\":[\"http://schema.mathworks.com/mf0/Connector/R2020b\"],\"version\":\"1.0\"}"
  TEMP_01 : Subsystem
  Thermal Mass of inside air : fl_lib/Thermal/Thermal Elements/Thermal Mass  mass_type=foundation.enum.constant_variable.constant  mass=P_M_AIR_HALL kg  sp_heat=P_CP_AIR J/(K*kg)  mass_min=1e-6 kg  num_ports=foundation.enum.numPorts2.one  m_specify=off  m_priority=High  m=1 kg  m_nominal_specify=off  m_nominal_unit=kg  m_nominal_value=1  T_specify=on  T_priority=High  T=T_INIT_BDR degC  T_nominal_specify=off  T_nominal_unit=K  T_nominal_value=1  Q_specify=off  Q_priority=None  Q=0 W  Q_nominal_specify=off  Q_nominal_unit=W  Q_nominal_value=1
  Wall (Hall<->Outside) : Subsystem
  Conn1 : PMIOPort  Side=Left
  T_HALL : Outport
  wires:
  TEMP_01/1(Sim) -> T_HALL/1
  [T_OUT] -> Outside Temperature/1(T_OUT)
  [T_ENV] -> Inside Enivornment Temperature/1(T_ENV)
  connections:
  TEMP_01/LConn1 -- Ceiling & Floor (Hall<->Above & Below)/RConn1 -- Conn1/RConn1 -- Wall (Hall<->Outside)/LConn1 -- Thermal Mass of inside air/LConn1
  Inside Enivornment Temperature/LConn1 -- Ceiling & Floor (Hall<->Above & Below)/LConn1
  Outside Temperature/LConn1 -- Wall (Hall<->Outside)/RConn1

== system Task_No6_Thermal/sub_House/Kitchen ==
  Ceiling & Floor (KIT<->Above & Below) : Subsystem
  Heat source human : Subsystem
  Inside Enivornment Temperature : Subsystem
      settings: PortSchema="{\"entries\":[{\"content\":{\"sides\":[{\"content\":{\"connectorIds\":[\"LConn1\"]},\"type\":\"ConnectorPlacement.EquallySpacedRectSide\",\"uuid\":\"d7207a88-d4d1-4eb1-8525-bfbf38cfed80\"},{\"content\":{\"connectorIds\":[\"In1\"],\"side\":\"RIGHT\"},\"type\":\"ConnectorPlacement.EquallySpacedRectSide\",\"uuid\":\"a5beddf3-616c-4e89-970e-855bf6dc3854\"},{\"content\":{\"side\":\"TOP\"},\"type\":\"ConnectorPlacement.EquallySpacedRectSide\",\"uuid\":\"3f9b2b25-be8a-4286-a049-e39ed58f5b46\"}]},\"type\":\"ConnectorPlacement.EquallySpacedConnector\",\"uuid\":\"525311df-b3f4-411a-b576-8112a1b0b63b\"}],\"packageUris\":[\"http://schema.mathworks.com/mf0/Connector/R2020b\"],\"version\":\"1.0\"}"
  Outside Temperature : Subsystem
      settings: PortSchema="{\"entries\":[{\"content\":{\"sides\":[{\"content\":{\"connectorIds\":[\"LConn1\"]},\"type\":\"ConnectorPlacement.EquallySpacedRectSide\",\"uuid\":\"d7207a88-d4d1-4eb1-8525-bfbf38cfed80\"},{\"content\":{\"connectorIds\":[\"In1\"],\"side\":\"RIGHT\"},\"type\":\"ConnectorPlacement.EquallySpacedRectSide\",\"uuid\":\"a5beddf3-616c-4e89-970e-855bf6dc3854\"},{\"content\":{\"side\":\"TOP\"},\"type\":\"ConnectorPlacement.EquallySpacedRectSide\",\"uuid\":\"3f9b2b25-be8a-4286-a049-e39ed58f5b46\"}]},\"type\":\"ConnectorPlacement.EquallySpacedConnector\",\"uuid\":\"525311df-b3f4-411a-b576-8112a1b0b63b\"}],\"packageUris\":[\"http://schema.mathworks.com/mf0/Connector/R2020b\"],\"version\":\"1.0\"}"
  SOLAR__WALL : Subsystem
  SOLAR__WINDOW : Subsystem
  TEMP_01 : Subsystem
  Thermal Mass of inside air : fl_lib/Thermal/Thermal Elements/Thermal Mass  mass_type=foundation.enum.constant_variable.constant  mass=P_M_AIR_KIT kg  sp_heat=P_CP_AIR J/(K*kg)  mass_min=1e-6 kg  num_ports=foundation.enum.numPorts2.one  m_specify=off  m_priority=High  m=1 kg  m_nominal_specify=off  m_nominal_unit=kg  m_nominal_value=1  T_specify=on  T_priority=High  T=T_INIT_BDR degC  T_nominal_specify=off  T_nominal_unit=K  T_nominal_value=1  Q_specify=off  Q_priority=None  Q=0 W  Q_nominal_specify=off  Q_nominal_unit=W  Q_nominal_value=1
  Wall (KIT<->Outside) : Subsystem
  Window (KIT<->Outside) : Subsystem
  Conn1 : PMIOPort  Side=Left
  T_KIT : Outport
  wires:
  TEMP_01/1(Sim) -> T_KIT/1
  [T_OUT] -> Outside Temperature/1(T_OUT)
  [T_ENV] -> Inside Enivornment Temperature/1(T_ENV)
  connections:
  Window (KIT<->Outside)/RConn1 -- Outside Temperature/LConn1 -- Wall (KIT<->Outside)/RConn2
  TEMP_01/LConn1 -- Heat source human/LConn1 -- Conn1/RConn1 -- Wall (KIT<->Outside)/LConn1 -- Thermal Mass of inside air/LConn1 -- Window (KIT<->Outside)/LConn1 -- Ceiling & Floor (KIT<->Above & Below)/RConn1
  Inside Enivornment Temperature/LConn1 -- Ceiling & Floor (KIT<->Above & Below)/LConn1
  SOLAR__WALL/LConn1 -- Wall (KIT<->Outside)/RConn1
  SOLAR__WINDOW/LConn1 -- Window (KIT<->Outside)/RConn2

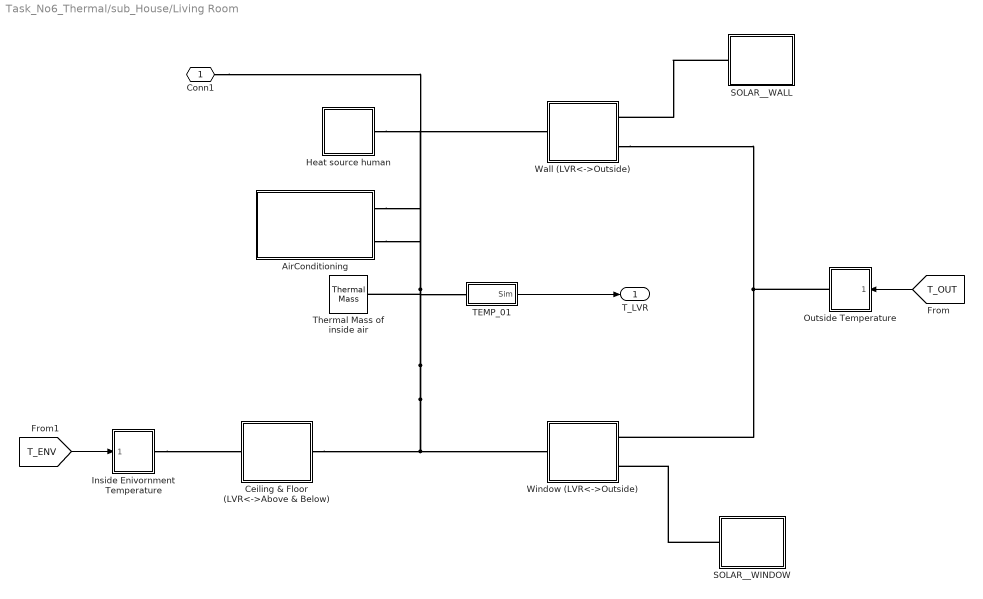
== system Task_No6_Thermal/sub_House/Living Room ==
  AirConditioning : Subsystem
  Ceiling & Floor (LVR<->Above & Below) : Subsystem
  Heat source human : Subsystem
  Inside Enivornment Temperature : Subsystem
      settings: PortSchema="{\"entries\":[{\"content\":{\"sides\":[{\"content\":{\"connectorIds\":[\"LConn1\"]},\"type\":\"ConnectorPlacement.EquallySpacedRectSide\",\"uuid\":\"d7207a88-d4d1-4eb1-8525-bfbf38cfed80\"},{\"content\":{\"connectorIds\":[\"In1\"],\"side\":\"RIGHT\"},\"type\":\"ConnectorPlacement.EquallySpacedRectSide\",\"uuid\":\"a5beddf3-616c-4e89-970e-855bf6dc3854\"},{\"content\":{\"side\":\"TOP\"},\"type\":\"ConnectorPlacement.EquallySpacedRectSide\",\"uuid\":\"3f9b2b25-be8a-4286-a049-e39ed58f5b46\"}]},\"type\":\"ConnectorPlacement.EquallySpacedConnector\",\"uuid\":\"525311df-b3f4-411a-b576-8112a1b0b63b\"}],\"packageUris\":[\"http://schema.mathworks.com/mf0/Connector/R2020b\"],\"version\":\"1.0\"}"
  Outside Temperature : Subsystem
      settings: PortSchema="{\"entries\":[{\"content\":{\"sides\":[{\"content\":{\"connectorIds\":[\"LConn1\"]},\"type\":\"ConnectorPlacement.EquallySpacedRectSide\",\"uuid\":\"d7207a88-d4d1-4eb1-8525-bfbf38cfed80\"},{\"content\":{\"connectorIds\":[\"In1\"],\"side\":\"RIGHT\"},\"type\":\"ConnectorPlacement.EquallySpacedRectSide\",\"uuid\":\"a5beddf3-616c-4e89-970e-855bf6dc3854\"},{\"content\":{\"side\":\"TOP\"},\"type\":\"ConnectorPlacement.EquallySpacedRectSide\",\"uuid\":\"3f9b2b25-be8a-4286-a049-e39ed58f5b46\"}]},\"type\":\"ConnectorPlacement.EquallySpacedConnector\",\"uuid\":\"525311df-b3f4-411a-b576-8112a1b0b63b\"}],\"packageUris\":[\"http://schema.mathworks.com/mf0/Connector/R2020b\"],\"version\":\"1.0\"}"
  SOLAR__WALL : Subsystem
  SOLAR__WINDOW : Subsystem
  TEMP_01 : Subsystem
  Thermal Mass of inside air : fl_lib/Thermal/Thermal Elements/Thermal Mass  mass_type=foundation.enum.constant_variable.constant  mass=P_M_AIR_LVR kg  sp_heat=P_CP_AIR J/(K*kg)  mass_min=1e-6 kg  num_ports=foundation.enum.numPorts2.one  m_specify=off  m_priority=High  m=1 kg  m_nominal_specify=off  m_nominal_unit=kg  m_nominal_value=1  T_specify=on  T_priority=High  T=T_INIT_BDR degC  T_nominal_specify=off  T_nominal_unit=K  T_nominal_value=1  Q_specify=off  Q_priority=None  Q=0 W  Q_nominal_specify=off  Q_nominal_unit=W  Q_nominal_value=1
  Wall (LVR<->Outside) : Subsystem
  Window (LVR<->Outside) : Subsystem
  Conn1 : PMIOPort  Side=Left
  T_LVR : Outport
  wires:
  TEMP_01/1(Sim) -> T_LVR/1
  [T_OUT] -> Outside Temperature/1(T_OUT)
  [T_ENV] -> Inside Enivornment Temperature/1(T_ENV)
  connections:
  Inside Enivornment Temperature/LConn1 -- Ceiling & Floor (LVR<->Above & Below)/LConn1
  Ceiling & Floor (LVR<->Above & Below)/RConn1 -- Window (LVR<->Outside)/LConn1 -- Thermal Mass of inside air/LConn1 -- AirConditioning/RConn2 -- AirConditioning/RConn1 -- Heat source human/LConn1 -- Wall (LVR<->Outside)/LConn1 -- Conn1/RConn1 -- TEMP_01/LConn1
  Wall (LVR<->Outside)/RConn2 -- Outside Temperature/LConn1 -- Window (LVR<->Outside)/RConn1
  SOLAR__WALL/LConn1 -- Wall (LVR<->Outside)/RConn1
  SOLAR__WINDOW/LConn1 -- Window (LVR<->Outside)/RConn2

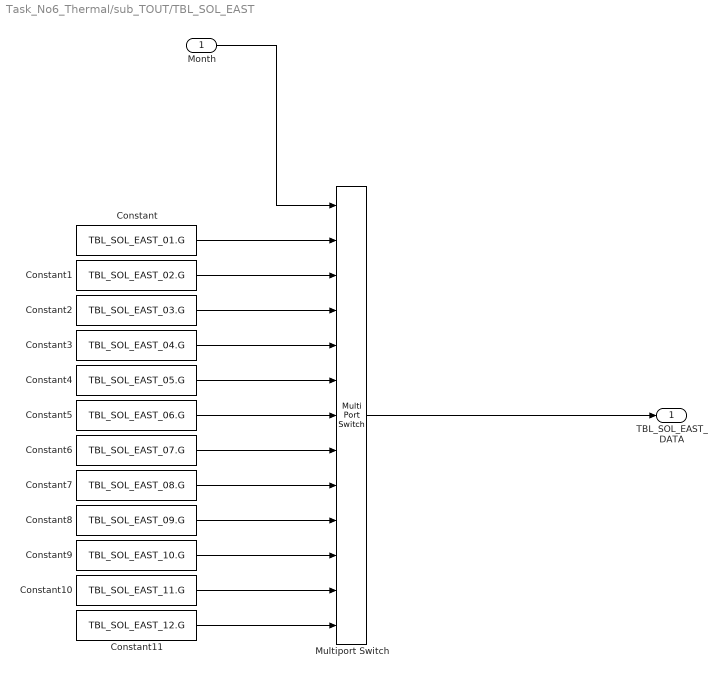
== system Task_No6_Thermal/sub_TOUT/TBL_SOL_EAST ==
  Month : Inport
  Constant : Constant  Value=TBL_SOL_EAST_01.G
  Constant1 : Constant  Value=TBL_SOL_EAST_02.G
  Constant10 : Constant  Value=TBL_SOL_EAST_11.G
  Constant11 : Constant  Value=TBL_SOL_EAST_12.G
  Constant2 : Constant  Value=TBL_SOL_EAST_03.G
  Constant3 : Constant  Value=TBL_SOL_EAST_04.G
  Constant4 : Constant  Value=TBL_SOL_EAST_05.G
  Constant5 : Constant  Value=TBL_SOL_EAST_06.G
  Constant6 : Constant  Value=TBL_SOL_EAST_07.G
  Constant7 : Constant  Value=TBL_SOL_EAST_08.G
  Constant8 : Constant  Value=TBL_SOL_EAST_09.G
  Constant9 : Constant  Value=TBL_SOL_EAST_10.G
  Multiport Switch : MultiPortSwitch  Inputs=12  SaturateOnIntegerOverflow=off  InputSameDT=off
  TBL_SOL_EAST_DATA : Outport
  wires:
  Constant1/1 -> Multiport Switch/3
  Constant5/1 -> Multiport Switch/7
  Constant6/1 -> Multiport Switch/8
  Constant3/1 -> Multiport Switch/5
  Multiport Switch/1 -> TBL_SOL_EAST_DATA/1
  Constant11/1 -> Multiport Switch/13
  Constant/1 -> Multiport Switch/2
  Constant2/1 -> Multiport Switch/4
  Constant7/1 -> Multiport Switch/9
  Constant4/1 -> Multiport Switch/6
  Constant10/1 -> Multiport Switch/12
  Constant9/1 -> Multiport Switch/11
  Constant8/1 -> Multiport Switch/10
  Month/1 -> Multiport Switch/1

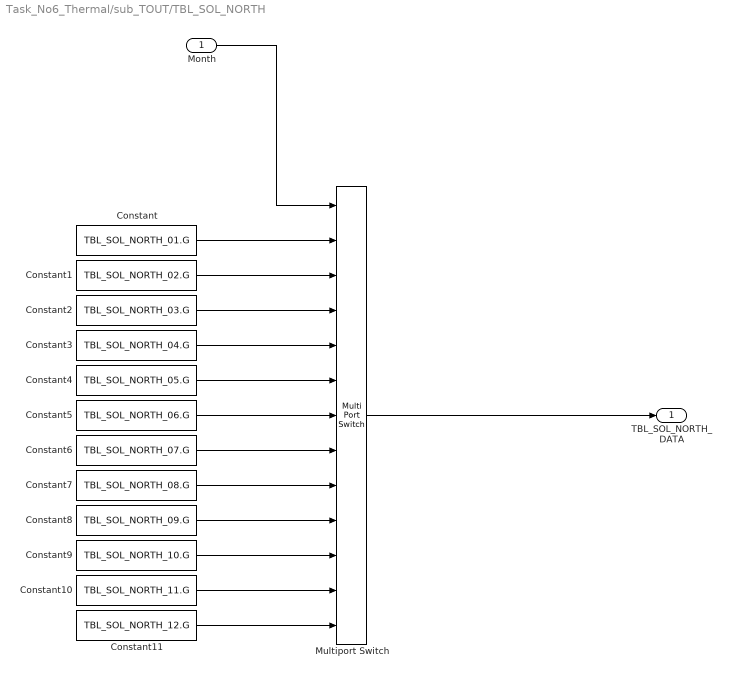
== system Task_No6_Thermal/sub_TOUT/TBL_SOL_NORTH ==
  Month : Inport
  Constant : Constant  Value=TBL_SOL_NORTH_01.G
  Constant1 : Constant  Value=TBL_SOL_NORTH_02.G
  Constant10 : Constant  Value=TBL_SOL_NORTH_11.G
  Constant11 : Constant  Value=TBL_SOL_NORTH_12.G
  Constant2 : Constant  Value=TBL_SOL_NORTH_03.G
  Constant3 : Constant  Value=TBL_SOL_NORTH_04.G
  Constant4 : Constant  Value=TBL_SOL_NORTH_05.G
  Constant5 : Constant  Value=TBL_SOL_NORTH_06.G
  Constant6 : Constant  Value=TBL_SOL_NORTH_07.G
  Constant7 : Constant  Value=TBL_SOL_NORTH_08.G
  Constant8 : Constant  Value=TBL_SOL_NORTH_09.G
  Constant9 : Constant  Value=TBL_SOL_NORTH_10.G
  Multiport Switch : MultiPortSwitch  Inputs=12  SaturateOnIntegerOverflow=off  InputSameDT=off
  TBL_SOL_NORTH_DATA : Outport
  wires:
  Month/1 -> Multiport Switch/1
  Constant8/1 -> Multiport Switch/10
  Constant9/1 -> Multiport Switch/11
  Constant10/1 -> Multiport Switch/12
  Constant4/1 -> Multiport Switch/6
  Constant7/1 -> Multiport Switch/9
  Constant2/1 -> Multiport Switch/4
  Constant/1 -> Multiport Switch/2
  Constant11/1 -> Multiport Switch/13
  Multiport Switch/1 -> TBL_SOL_NORTH_DATA/1
  Constant3/1 -> Multiport Switch/5
  Constant6/1 -> Multiport Switch/8
  Constant5/1 -> Multiport Switch/7
  Constant1/1 -> Multiport Switch/3

== system Task_No6_Thermal/sub_TOUT/TBL_SOL_SOUTH ==
  Month : Inport
  Constant{,1..11} (12 alike) : Constant  Value=TBL_SOL_SOUTH_01.G
  Multiport Switch : MultiPortSwitch  Inputs=12  SaturateOnIntegerOverflow=off  InputSameDT=off
  TBL_SOL_SOUTH_DATA : Outport
  wires:
  Constant1/1 -> Multiport Switch/3
  Constant5/1 -> Multiport Switch/7
  Constant6/1 -> Multiport Switch/8
  Constant3/1 -> Multiport Switch/5
  Multiport Switch/1 -> TBL_SOL_SOUTH_DATA/1
  Constant11/1 -> Multiport Switch/13
  Constant/1 -> Multiport Switch/2
  Constant2/1 -> Multiport Switch/4
  Constant7/1 -> Multiport Switch/9
  Constant4/1 -> Multiport Switch/6
  Constant10/1 -> Multiport Switch/12
  Constant9/1 -> Multiport Switch/11
  Constant8/1 -> Multiport Switch/10
  Month/1 -> Multiport Switch/1

== system Task_No6_Thermal/sub_House/Bathroom/Ceiling & Floor (Bath<->Above & Below) ==
  Ceiling-InAir : fl_lib/Thermal/Thermal Elements/Thermal Resistance  resistance=1/(U_CEIL*P_AREA_BATH) K/W  T_specify=off  T_priority=None  T=0 K  T_nominal_specify=off  T_nominal_unit=K  T_nominal_value=1  Q_specify=off  Q_priority=None  Q=0 W  Q_nominal_specify=off  Q_nominal_unit=W  Q_nominal_value=1
  Floor-InAir : fl_lib/Thermal/Thermal Elements/Thermal Resistance  resistance=1/(U_CEIL*P_AREA_BATH) K/W  T_specify=off  T_priority=None  T=0 K  T_nominal_specify=off  T_nominal_unit=K  T_nominal_value=1  Q_specify=off  Q_priority=None  Q=0 W  Q_nominal_specify=off  Q_nominal_unit=W  Q_nominal_value=1
  Conn1 : PMIOPort  Side=Left
  Conn2 : PMIOPort  Port=2  Side=Right
  connections:
  Floor-InAir/RConn1 -- Ceiling-InAir/RConn1 -- Conn2/RConn1
  Floor-InAir/LConn1 -- Ceiling-InAir/LConn1 -- Conn1/RConn1

== system Task_No6_Thermal/sub_House/Bathroom/Inside Enivornment Temperature ==
  T_ENV : Inport
  Constant2 : Constant  Value=Conv_C_to_K
  Controlled Temperature Source : fl_lib/Thermal/Thermal Sources/Controlled Temperature Source
  Simulink-PS Converter1 : nesl_utility/Simulink-PS Converter  PhysicalDomain=network_engine_domain  SubClassName=ps_input  LeftPortType=input  RightPortType=output  PseudoPeriodic=off  Frequencies=[]  NoiseDistribution=none  NoiseParameters=[]  Unit=1  AffineConversion=off  FilteringAndDerivatives=provide  SimscapeFilterOrder=1  InputFilterTimeConstant=0.001  UdotUserProvided=0
  Sum : Sum  Inputs=|++
  Thermal Reference1 : fl_lib/Thermal/Thermal Elements/Thermal Reference
  Conn1 : PMIOPort  Side=Left
  wires:
  T_ENV/1 -> Sum/1
  Constant2/1 -> Sum/2
  Sum/1 -> Simulink-PS Converter1/1
  connections:
  Controlled Temperature Source/LConn1 -- Conn1/RConn1
  Simulink-PS Converter1/RConn1 -- Controlled Temperature Source/RConn1
  Thermal Reference1/LConn1 -- Controlled Temperature Source/RConn2

== system Task_No6_Thermal/sub_House/Bathroom/Outside Temperature ==
  T_OUT : Inport
  Constant2 : Constant  Value=Conv_C_to_K
  Controlled Temperature Source : fl_lib/Thermal/Thermal Sources/Controlled Temperature Source
  Simulink-PS Converter1 : nesl_utility/Simulink-PS Converter  PhysicalDomain=network_engine_domain  SubClassName=ps_input  LeftPortType=input  RightPortType=output  PseudoPeriodic=off  Frequencies=[]  NoiseDistribution=none  NoiseParameters=[]  Unit=1  AffineConversion=off  FilteringAndDerivatives=provide  SimscapeFilterOrder=1  InputFilterTimeConstant=0.001  UdotUserProvided=0
  Sum : Sum  Inputs=|++
  Thermal Reference1 : fl_lib/Thermal/Thermal Elements/Thermal Reference
  Conn1 : PMIOPort  Side=Left
  wires:
  Sum/1 -> Simulink-PS Converter1/1
  Constant2/1 -> Sum/2
  T_OUT/1 -> Sum/1
  connections:
  Thermal Reference1/LConn1 -- Controlled Temperature Source/RConn2
  Simulink-PS Converter1/RConn1 -- Controlled Temperature Source/RConn1
  Controlled Temperature Source/LConn1 -- Conn1/RConn1

== system Task_No6_Thermal/sub_House/Bathroom/SOLAR__WALL ==
  Add : Sum
  Constant : Constant  Value=P_AREA_NORTH_WALL_BATH
  Constant1 : Constant  Value=P_EM_WALL
  Constant2 : Constant  Value=P_AREA_EAST_WALL_BATH
  Constant3 : Constant  Value=P_EM_WALL
  Controlled Heat Flow Rate Source : fl_lib/Thermal/Thermal Sources/Controlled Heat Flow Rate Source
  Product : Product  Inputs=3
  Product1 : Product  Inputs=3
  Simulink-PS Converter : nesl_utility/Simulink-PS Converter  PhysicalDomain=network_engine_domain  SubClassName=ps_input  LeftPortType=input  RightPortType=output  PseudoPeriodic=off  Frequencies=[]  NoiseDistribution=none  NoiseParameters=[]  Unit=1  AffineConversion=off  FilteringAndDerivatives=provide  SimscapeFilterOrder=1  InputFilterTimeConstant=0.001  UdotUserProvided=0
  Thermal Reference : fl_lib/Thermal/Thermal Elements/Thermal Reference
  Conn1 : PMIOPort  Side=Left
  wires:
  Constant/1 -> Product/2
  Constant1/1 -> Product/1
  [SOL_NORTH] -> Product/3
  Product/1 -> Add/1
  Constant3/1 -> Product1/1
  [SOL_EAST] -> Product1/3
  Constant2/1 -> Product1/2
  Add/1 -> Simulink-PS Converter/1
  Product1/1 -> Add/2
  connections:
  Controlled Heat Flow Rate Source/LConn1 -- Conn1/RConn1
  Simulink-PS Converter/RConn1 -- Controlled Heat Flow Rate Source/RConn1
  Thermal Reference/LConn1 -- Controlled Heat Flow Rate Source/RConn2

== system Task_No6_Thermal/sub_House/Bathroom/SOLAR__WINDOW ==
  Constant : Constant  Value=P_AREA_WIN_BATH
  Constant1 : Constant  Value=P_EM_GLASS
  Controlled Heat Flow Rate Source : fl_lib/Thermal/Thermal Sources/Controlled Heat Flow Rate Source
  Product : Product  Inputs=3
  Simulink-PS Converter : nesl_utility/Simulink-PS Converter  PhysicalDomain=network_engine_domain  SubClassName=ps_input  LeftPortType=input  RightPortType=output  PseudoPeriodic=off  Frequencies=[]  NoiseDistribution=none  NoiseParameters=[]  Unit=1  AffineConversion=off  FilteringAndDerivatives=provide  SimscapeFilterOrder=1  InputFilterTimeConstant=0.001  UdotUserProvided=0
  Thermal Reference : fl_lib/Thermal/Thermal Elements/Thermal Reference
  Conn1 : PMIOPort  Side=Left
  wires:
  Product/1 -> Simulink-PS Converter/1
  [SOL_EAST] -> Product/3
  Constant1/1 -> Product/1
  Constant/1 -> Product/2
  connections:
  Thermal Reference/LConn1 -- Controlled Heat Flow Rate Source/RConn2
  Simulink-PS Converter/RConn1 -- Controlled Heat Flow Rate Source/RConn1
  Controlled Heat Flow Rate Source/LConn1 -- Conn1/RConn1

== system Task_No6_Thermal/sub_House/Bathroom/TEMP_01 ==
  Constant2 : Constant  Value=Conv_C_to_K
  PS-Simulink Converter : nesl_utility/PS-Simulink Converter  PhysicalDomain=network_engine_domain  SubClassName=ps_output  LeftPortType=input  RightPortType=output  PseudoPeriodic=off  Frequencies=[]  VectorFormat=inherit  Unit=inherit  AffineConversion=off
  Sum : Sum  Inputs=|+-
  Temperature Sensor : fl_lib/Thermal/Thermal Sensors/Temperature Sensor  temperature_measure=foundation.enum.MeasurementReference.difference
  Thermal Reference2 : fl_lib/Thermal/Thermal Elements/Thermal Reference
  PS : PMIOPort  Side=Left
  Sim : Outport
  wires:
  Sum/1 -> Sim/1
  PS-Simulink Converter/1 -> Sum/1
  Constant2/1 -> Sum/2
  connections:
  Thermal Reference2/LConn1 -- Temperature Sensor/RConn1
  PS-Simulink Converter/LConn1 -- Temperature Sensor/RConn2
  PS/RConn1 -- Temperature Sensor/LConn1

== system Task_No6_Thermal/sub_House/Bathroom/Wall (Bath<->Outside) ==
  InAir-Wall : fl_lib/Thermal/Thermal Elements/Thermal Resistance  resistance=1/(U_WALL*P_AREA_OUTER_WALL_BATH)/2 K/W  T_specify=off  T_priority=None  T=0 K  T_nominal_specify=off  T_nominal_unit=K  T_nominal_value=1  Q_specify=off  Q_priority=None  Q=0 W  Q_nominal_specify=off  Q_nominal_unit=W  Q_nominal_value=1
  Thermal Mass of wall : fl_lib/Thermal/Thermal Elements/Thermal Mass  mass_type=foundation.enum.constant_variable.constant  mass=P_AREA_OUTER_WALL_BATH*(P_THICK_BRICK*P_DENSITY_BRICK+P_THICK_PUR*P_DENSITY_PUR) kg  sp_heat=P_CP_WALL J/(K*kg)  mass_min=1e-6 kg  num_ports=foundation.enum.numPorts2.one  m_specify=off  m_priority=High  m=1 kg  m_nominal_specify=off  m_nominal_unit=kg  m_nominal_value=1  T_specify=on  T_priority=High  T=T_INIT_BDR degC  T_nominal_specify=off  T_nominal_unit=K  T_nominal_value=1  Q_specify=off  Q_priority=None  Q=0 W  Q_nominal_specify=off  Q_nominal_unit=W  Q_nominal_value=1
  Wall-OutAir : fl_lib/Thermal/Thermal Elements/Thermal Resistance  resistance=1/(U_WALL*P_AREA_OUTER_WALL_BATH)/2 K/W  T_specify=off  T_priority=None  T=0 K  T_nominal_specify=off  T_nominal_unit=K  T_nominal_value=1  Q_specify=off  Q_priority=None  Q=0 W  Q_nominal_specify=off  Q_nominal_unit=W  Q_nominal_value=1
  Conn1 : PMIOPort  Side=Left
  Conn3 : PMIOPort  Port=2  Side=Right
  Conn2 : PMIOPort  Port=3  Side=Right
  connections:
  Conn1/RConn1 -- InAir-Wall/LConn1
  InAir-Wall/RConn1 -- Conn3/RConn1 -- Thermal Mass of wall/LConn1 -- Wall-OutAir/LConn1
  Wall-OutAir/RConn1 -- Conn2/RConn1

== system Task_No6_Thermal/sub_House/Bathroom/Window (Bath<->Outside) ==
  InAir-Window : fl_lib/Thermal/Thermal Elements/Thermal Resistance  resistance=1/(U_WINDOW*P_AREA_WIN_BATH)/2 K/W  T_specify=off  T_priority=None  T=0 K  T_nominal_specify=off  T_nominal_unit=K  T_nominal_value=1  Q_specify=off  Q_priority=None  Q=0 W  Q_nominal_specify=off  Q_nominal_unit=W  Q_nominal_value=1
  Thermal Mass of window : fl_lib/Thermal/Thermal Elements/Thermal Mass  mass_type=foundation.enum.constant_variable.constant  mass=P_M_WINDOW_SPEC*P_AREA_WIN_BATH kg  sp_heat=P_CP_GLASS J/(K*kg)  mass_min=1e-6 kg  num_ports=foundation.enum.numPorts2.one  m_specify=off  m_priority=High  m=1 kg  m_nominal_specify=off  m_nominal_unit=kg  m_nominal_value=1  T_specify=on  T_priority=High  T=T_INIT_BDR degC  T_nominal_specify=off  T_nominal_unit=K  T_nominal_value=1  Q_specify=off  Q_priority=None  Q=0 W  Q_nominal_specify=off  Q_nominal_unit=W  Q_nominal_value=1
  Window-OutAir : fl_lib/Thermal/Thermal Elements/Thermal Resistance  resistance=1/(U_WINDOW*P_AREA_WIN_BATH)/2 K/W  T_specify=off  T_priority=None  T=0 K  T_nominal_specify=off  T_nominal_unit=K  T_nominal_value=1  Q_specify=off  Q_priority=None  Q=0 W  Q_nominal_specify=off  Q_nominal_unit=W  Q_nominal_value=1
  Conn1 : PMIOPort  Side=Right
  Conn2 : PMIOPort  Port=2  Side=Left
  Conn3 : PMIOPort  Port=3  Side=Right
  connections:
  Thermal Mass of window/LConn1 -- Conn3/RConn1 -- Window-OutAir/LConn1 -- InAir-Window/RConn1
  Conn1/RConn1 -- Window-OutAir/RConn1
  Conn2/RConn1 -- InAir-Window/LConn1
